simulink model "Longitudinal_new"  (R2025b)
settings: Solver=VariableStepAuto  StartTime=0.0  StopTime=5  MaxStep=0.001  RelTol=1e-3
undefined symbols (not defined in the file): car, rad, s, Tau_1, Tau_2, Tau_3, Tau_4, Tau_EM, tyre
libraries: aerolibconvert2 x7, simulink x4, autolibcoupling x2
(part 3 of 3)

== matlab function Longitudinal_new/longitudinal dynamics/Kinematics/FL/Front Left Tyre ==
  data: car input; wheel_travel_FL output; IR_FL input; AD_FL input; Fz_FL input; h_ground_FL output; delta_Fz input; delta_z_tyre_FL output; a input
function [wheel_travel_FL, h_ground_FL, delta_z_tyre_FL] = kinematics(car, IR_FL, AD_FL, Fz_FL, delta_Fz, a)

delta_z_tyre_FL = Fz_FL / car.k_tyre/1000; % tyre vertical stiffness - kz_tyre - for front and rear tyres, look at buses
k_spring_ground_FL = (car.k_spring_front * IR_FL^2) + car.k_flexure;

if a > 0 % under acceleration
    delta_z_spring_FL = Fz_FL / k_spring_ground_FL; % front axle
else % under braking
    delta_z_spring_FL = (Fz_FL - delta_Fz) / k_spring_ground_FL + delta_Fz * ((1-AD_FL/100)/k_spring_ground_FL) ; % front axle
end

%wheel center movement only due to spring deflection at ground. 
%to be used in the kineamtics block (camber, antidive, ir,...)
wheel_travel_FL = delta_z_spring_FL - car.z0_spring_front; % if negative it is bounce

%to be used to find the new height of the car from the ground
jounce_FL = delta_z_tyre_FL + delta_z_spring_FL - car.z0_front;
h_ground_FL = car.h0_ground_front - jounce_FL;

== matlab function Longitudinal_new/longitudinal dynamics/slip_tyres/FR ==
  data: delta_Fx_front input; delta_z_tyre_FR input; w_dot_slip_FR output; car input
function w_dot_slip_FR  = slip(delta_Fx_front, delta_z_tyre_FR, car)


    w_dot_slip_FR = (delta_Fx_front * (car.R - delta_z_tyre_FR)) / car.J_f; %rad/s^2

== matlab function Longitudinal_new/Tyres1/Rear Left ==
  data: car input; Fx_RL output; SR input; Fz input; camber input
function Fx_RL = fcn(car,SR,Fz,camber)

% PAC2002 puro longitudinale (Fx vs k)

     Fz0 = car.tyre_Fz0;
     if Fz0 == 0, Fz0 = max(1, Fz); end
    dfz = (Fz - Fz0)/Fz0;

    pi0 = car.tyre_pi0;  % Pa nominale
    dpi = (car.tyre_pressure_rear - pi0)/pi0;
    
Cx1 = car.tyre_Cx1;
Dx1 = car.tyre_Dx1;
Dx2 = car.tyre_Dx2;
Dx3 = car.tyre_Dx3;
Ex1 = car.tyre_Ex1;
Ex2 = car.tyre_Ex2;
Ex3 = car.tyre_Ex3;
Ex4 = car.tyre_Ex4;
Kx1 = car.tyre_Kx1;
Kx2 = car.tyre_Kx2;
Kx3 = car.tyre_Kx3;
Hx1 = car.tyre_Hx1;
Hx2 = car.tyre_Hx2;
Vx1 = car.tyre_Vx1;
Vx2 = car.tyre_Vx2;
px1 = car.tyre_px1;
px2 = car.tyre_px2;
px3 = car.tyre_px3;
px4 = car.tyre_px4;
% lmux = car.tyre_lmux;


    gamma = camber*pi/180;
    mu = (Dx1 + Dx2*dfz) * (1 - Dx3*(gamma^2)) * (1 + px3*dpi + px4*dpi^2)*car.scale_factor;
    % mu = 1.4;

    D = mu * Fz;
    C = Cx1;
    K = Fz * (Kx1 + Kx2*dfz) * exp(Kx3*dfz) * (1 + px1*dpi + px2*dpi^2);
    B = K / (C*D + eps);

    SH = Hx1 + Hx2*dfz;
    SR  = SR + SH;

    E  = (Ex1 + Ex2*dfz + Ex3*dfz^2) * (1 - Ex4*sign(SR));
    SV = Fz * (Vx1 + Vx2*dfz);

    Fx0 = D * sin( C * atan( B*SR - E*(B*SR - atan(B*SR)) ) );
    Fx_RL = Fx0 + SV;

== matlab function Longitudinal_new/Tyres1/Rear Right ==
  data: car input; Fx_RR output; SR input; Fz input; camber input
function Fx_RR = fcn(car,SR,Fz,camber)

% PAC2002 puro longitudinale (Fx vs k)

     Fz0 = car.tyre_Fz0;
     if Fz0 == 0, Fz0 = max(1, Fz); end
    dfz = (Fz - Fz0)/Fz0;

    pi0 = car.tyre_pi0;  % Pa nominale
    dpi = (car.tyre_pressure_rear - pi0)/pi0;
    
Cx1 = car.tyre_Cx1;
Dx1 = car.tyre_Dx1;
Dx2 = car.tyre_Dx2;
Dx3 = car.tyre_Dx3;
Ex1 = car.tyre_Ex1;
Ex2 = car.tyre_Ex2;
Ex3 = car.tyre_Ex3;
Ex4 = car.tyre_Ex4;
Kx1 = car.tyre_Kx1;
Kx2 = car.tyre_Kx2;
Kx3 = car.tyre_Kx3;
Hx1 = car.tyre_Hx1;
Hx2 = car.tyre_Hx2;
Vx1 = car.tyre_Vx1;
Vx2 = car.tyre_Vx2;
px1 = car.tyre_px1;
px2 = car.tyre_px2;
px3 = car.tyre_px3;
px4 = car.tyre_px4;
% lmux = car.tyre_lmux;


    gamma = camber*pi/180;
    mu = (Dx1 + Dx2*dfz) * (1 - Dx3*(gamma^2)) * (1 + px3*dpi + px4*dpi^2)*car.scale_factor;
    % mu = 1.4;

    D = mu * Fz;
    C = Cx1;
    K = Fz * (Kx1 + Kx2*dfz) * exp(Kx3*dfz) * (1 + px1*dpi + px2*dpi^2);
    B = K / (C*D + eps);

    SH = Hx1 + Hx2*dfz;
    SR  = SR + SH;

    E  = (Ex1 + Ex2*dfz + Ex3*dfz^2) * (1 - Ex4*sign(SR));
    SV = Fz * (Vx1 + Vx2*dfz);

    Fx0 = D * sin( C * atan( B*SR - E*(B*SR - atan(B*SR)) ) );
    Fx_RR = Fx0 + SV;

== matlab function Longitudinal_new/Powertrain/MATLAB Function ==
  settings: updateMethod=DISCRETE
  data: T_RL_in input; T_RR_in input; T_RL_out output; trigger input; T_RR_out output; time input
function [T_RL_out,T_RR_out] = fcn(T_RL_in, T_RR_in, trigger, time)

persistent t_start is_active prev_trigger
if isempty(t_start)
    t_start     = 0;
    is_active   = false;
    prev_trigger = 0;
end

% Rileva fronte di salita del trigger
if trigger == 1 && prev_trigger == 0
    t_start   = time;     % istante in cui parte il taglio coppia
    is_active = true;
end

% Disattiva dopo 0.15 s
if is_active && (time - t_start >= 0.15)
    is_active = false;
end

% Aggiorna trigger precedente
prev_trigger = trigger;

% Logica di uscita
if is_active
    T_RL_out = 0;
    T_RR_out = 0;
else
    T_RL_out = T_RL_in;
    T_RR_out = T_RR_in;
end
end

== matlab function Longitudinal_new/Powertrain/Clutch/MATLAB Function ==
  data: threshold input; w_out output; w_rear_in input; w_rear_out output
function [w_out, w_rear_out] = fcn(threshold, w_rear_in)

if w_rear_in < threshold
    w_out=threshold;
    w_rear_out=0;
else
    w_out=0;
    w_rear_out=w_rear_in;
end

== matlab function Longitudinal_new/longitudinal dynamics/Jr/MATLAB Function ==
  data: gear input; Jr_tot output; car input
function Jr_tot  = Jr(gear, car)

if gear == 1 
    Jr_tot = car.Jr_tot_1;
elseif gear == 2 
    Jr_tot = car.Jr_tot_2;
elseif gear == 3 
    Jr_tot = car.Jr_tot_3;
elseif gear == 4
    Jr_tot = car.Jr_tot_4;
else  
    Jr_tot = car.Jr_tot_0;
end

== matlab function Longitudinal_new/Powertrain/Clutch/MATLAB Function1 ==
  data: threshold input; w_out output; w_rear_in input; w_rear_out output
function [w_out, w_rear_out] = fcn(threshold, w_rear_in)

persistent isZero   % flag that stays true once threshold is reached

% Initialize the flag the first time the function is called
if isempty(isZero)
    isZero = false;
end

if w_rear_in >= threshold
    isZero = true;
end

% Output logic
if isZero
    w_out = 0;
    w_rear_out = w_rear_in;
else
    w_out = threshold;
    w_rear_out = 0;
end

end

== matlab function Longitudinal_new/Powertrain1/Driver model - gear selection1/MATLAB Function3 ==
  settings: updateMethod=DISCRETE
  data: gear_trigger output; car input; gear_out output; v input
function [gear_trigger, gear_out] = change_gear(car, v)

    persistent gear
    if isempty(gear)
        gear = 2;      % start in 2nd
    end

    R = car.R; %

    % thresholds
    v_thresh_up   = [0, 24.9444, 45];   % 1-2, 2-3, 3-4
    % v_thresh_down = [0, 15, 15];          % 2-1, 3-2, 4-3, i numeri sono a caso quindi da cambiare

    tau      = [13.8304, 9.9320, 8.5118, 7.4490];
    nGearMax = numel(tau);

    gear_trigger = 0;
    old_gear     = gear;   % save old gear
    gear_out     = old_gear;

    % - UPSHIFT
    if old_gear < nGearMax && v >= v_thresh_up(old_gear)
        gear = old_gear + 1;
        gear_trigger = 1;

    % % - DOWNSHIFT
    % elseif old_gear > 2 && v <= v_thresh_down(old_gear)
    %     gear = old_gear - 1;
    %     gear_trigger = -1;
    % end

    gear_out = gear;
end

== matlab function Longitudinal_new/longitudinal dynamics/Fx powertrain calculation/RR ==
  data: Fx_ICE_RR output; T input; T_b input; a input; Fz input; J_r input; car input; delta_z_tyre_RR input
function Fx_ICE_RR = fcn( T, T_b,a, Fz, J_r, car, delta_z_tyre_RR)

Fx_ICE_RR = ( T - T_b - Fz * car.delta - J_r * a / ( car.R - delta_z_tyre_RR ) ) / ( car.R - delta_z_tyre_RR ) ; %N; % J - parameter for each tyre - J_f & J_r

== matlab function Longitudinal_new/longitudinal dynamics/Fx powertrain calculation/FR ==
  data: Fx_EM_FR output; T input; T_b input; Fz input; a input; car input; delta_z_tyre_FR input
function Fx_EM_FR = fcn( T, T_b,Fz, a, car, delta_z_tyre_FR )

Fx_EM_FR = ( T - T_b - Fz * car.delta - car.J_f * a / ( car.R - delta_z_tyre_FR ) ) / ( car.R - delta_z_tyre_FR ) ; %N % J - parameter for each tyre - J_f & J_r

== matlab function Longitudinal_new/Tyres1/Front Left ==
  data: car input; Fx_FL output; SR input; Fz input; camber input
function Fx_FL = fcn(car,SR,Fz,camber)

% PAC2002 puro longitudinale (Fx vs k)

     Fz0 = car.tyre_Fz0;
     if Fz0 == 0, Fz0 = max(1, Fz); end
    dfz = (Fz - Fz0)/Fz0;

    pi0 = car.tyre_pi0;  % Pa nominale
    dpi = (car.tyre_pressure_front - pi0)/pi0;
    
Cx1 = car.tyre_Cx1;
Dx1 = car.tyre_Dx1;
Dx2 = car.tyre_Dx2;
Dx3 = car.tyre_Dx3;
Ex1 = car.tyre_Ex1;
Ex2 = car.tyre_Ex2;
Ex3 = car.tyre_Ex3;
Ex4 = car.tyre_Ex4;
Kx1 = car.tyre_Kx1;
Kx2 = car.tyre_Kx2;
Kx3 = car.tyre_Kx3;
Hx1 = car.tyre_Hx1;
Hx2 = car.tyre_Hx2;
Vx1 = car.tyre_Vx1;
Vx2 = car.tyre_Vx2;
px1 = car.tyre_px1;
px2 = car.tyre_px2;
px3 = car.tyre_px3;
px4 = car.tyre_px4;
% lmux = car.tyre_lmux;


    gamma = camber*pi/180;
    mu = (Dx1 + Dx2*dfz) * (1 - Dx3*(gamma^2)) * (1 + px3*dpi + px4*dpi^2)*car.scale_factor;
    % mu = 1.4;

    D = mu * Fz;
    C = Cx1;
    K = Fz * (Kx1 + Kx2*dfz) * exp(Kx3*dfz) * (1 + px1*dpi + px2*dpi^2);
    B = K / (C*D + eps);

    SH = Hx1 + Hx2*dfz;
    SR  = SR + SH;

    E  = (Ex1 + Ex2*dfz + Ex3*dfz^2) * (1 - Ex4*sign(SR));
    SV = Fz * (Vx1 + Vx2*dfz);

    Fx0 = D * sin( C * atan( B*SR - E*(B*SR - atan(B*SR)) ) );
    Fx_FL = Fx0 + SV;

== matlab function Longitudinal_new/longitudinal dynamics/Fx powertrain calculation/RL ==
  data: T input; T_b input; Fz input; a input; J_r input; car input; Fx_ICE_RL output; delta_z_tyre_RL input
function Fx_ICE_RL = fcn( T, T_b, Fz, a, J_r, car, delta_z_tyre_RL)

Fx_ICE_RL = ( T - T_b - Fz * car.delta - J_r * a / ( car.R - delta_z_tyre_RL ) ) / ( car.R - delta_z_tyre_RL ) ; %N % J - parameter for each tyre - J_f & J_r

== matlab function Longitudinal_new/longitudinal dynamics/delta_ Fx solver/RL ==
  data: Fx_ICE input; Fx_tyre input; delta_Fx_RL output
function delta_Fx_RL  = fcn(Fx_ICE, Fx_tyre)

delta_Fx_RL = Fx_ICE - Fx_tyre;

== matlab function Longitudinal_new/longitudinal dynamics/delta_ Fx solver/FR ==
  data: Fx_EM input; Fx_tyre input; delta_Fx_FR output
function delta_Fx_FR  = fcn(Fx_EM, Fx_tyre)

delta_Fx_FR = Fx_EM - Fx_tyre ;

== matlab function Longitudinal_new/longitudinal dynamics/delta_ Fx solver/FL ==
  data: Fx_EM input; Fx_tyre input; delta_Fx_FL output
function delta_Fx_FL  = fcn(Fx_EM, Fx_tyre)

delta_Fx_FL = Fx_EM - Fx_tyre;

== matlab function Longitudinal_new/Powertrain/Driver model - gear selection/MATLAB Function3 ==
  settings: updateMethod=DISCRETE
  data: gear_trigger output; car input; gear_out output; v input
function [gear_trigger, gear_out] = change_gear(car, v)

    persistent gear
    if isempty(gear)
        gear = 2;      % start in 2nd
    end

    R = car.R; %

    % thresholds
    v_thresh_up   = [0, 24.9444, 45];   % 1-2, 2-3, 3-4
    v_thresh_down = [0, 15, 15];          % 2-1, 3-2, 4-3, i numeri sono a caso quindi da cambiare

    tau      = [13.8304, 9.9320, 8.5118, 7.4490];
    nGearMax = numel(tau);

    gear_trigger = 0;
    old_gear     = gear;   % save old gear
    gear_out     = old_gear;

    % - UPSHIFT
    if old_gear < nGearMax && v >= v_thresh_up(old_gear)
        gear = old_gear + 1;
        gear_trigger = 1;

    % - DOWNSHIFT
    elseif old_gear > 2 && v <= v_thresh_down(old_gear)
        gear = old_gear - 1;
        gear_trigger = -1;
    end

    gear_out = gear;
end

== matlab function Longitudinal_new/longitudinal dynamics/slip_tyres/FL ==
  data: delta_Fx_front input; delta_z_tyre_FL input; w_dot_slip_FL output; car input
function w_dot_slip_FL  = slip(delta_Fx_front, delta_z_tyre_FL, car)

w_dot_slip_FL = delta_Fx_front * (car.R - delta_z_tyre_FL) / car.J_f;

== matlab function Longitudinal_new/longitudinal dynamics/slip_tyres/RL ==
  data: delta_Fx_rear input; w_dot_slip_RL output; delta_z_tyre_RL input; J_r input; car input
function w_dot_slip_RL  = slip(delta_Fx_rear, delta_z_tyre_RL, J_r, car)

w_dot_slip_RL = delta_Fx_rear * (car.R - delta_z_tyre_RL) / ( J_r );

== matlab function Longitudinal_new/Powertrain1/MATLAB Function2 ==
  data: w_ICE input; T_powertrain output; T_ICE input; w_rear input; T_clutch input; abs_w output
function [T_powertrain, abs_w] = Clutch(w_ICE, T_ICE, w_rear, T_clutch)

abs_w = w_ICE - w_rear;

if abs_w < 50
    T_powertrain = T_ICE;
else 
    T_powertrain = T_clutch;
end

== matlab function Longitudinal_new/Powertrain1/Clutch/MATLAB Function ==
  data: threshold input; w_out output; w_rear_in input; w_rear_out output
function [w_out, w_rear_out] = fcn(threshold, w_rear_in)

if w_rear_in < threshold
    w_out=threshold;
    w_rear_out=0;
else
    w_out=0;
    w_rear_out=w_rear_in;
end

== matlab function Longitudinal_new/Powertrain1/Clutch/MATLAB Function1 ==
  data: threshold input; w_out output; w_rear_in input; w_rear_out output
function [w_out, w_rear_out] = fcn(threshold, w_rear_in)

persistent isZero   % flag that stays true once threshold is reached

% Initialize the flag the first time the function is called
if isempty(isZero)
    isZero = false;
end

if w_rear_in >= threshold
    isZero = true;
end

% Output logic
if isZero
    w_out = 0;
    w_rear_out = w_rear_in;
else
    w_out = threshold;
    w_rear_out = 0;
end

end

== matlab function Longitudinal_new/longitudinal dynamics/Fx equilibrium ==
  data: Drag output; Fz_FL output; a input; Fz_RR output; Fz_RL output; Fz_FR output; delta_Fz output; v input; Cx input; Cz input; delta_wb_front input; delta_wb_rear input; Jr_tot input; car input
function [Drag, Fz_FL, Fz_RR, Fz_RL, Fz_FR, delta_Fz] = fx_equilibrium(a, v, Cx, Cz, delta_wb_front, delta_wb_rear, Jr_tot, car)

wb = car.wb0 + delta_wb_front + delta_wb_rear; %m

Downforce = 0.5 * car.rho * Cz * car.frontal_area * v ^ 2; % downforce N
Drag = 0.5 * car.rho * Cx * car.frontal_area * v ^ 2; % drag N
M_aero = Drag * (car.h_cp - car.h_cog) - Downforce * (car.lf - car.x_cp); %Nm

delta_Fz = car.m * a * car.h_cog / wb + Drag * car.h_cog / wb + M_aero / wb; %N
delta_Fz=delta_Fz/2;
%J_f è di una singola ruota
%J_r totale da ruota a motore ICE
Fz_front = -(car.m * a + Drag) * car.h_cog / wb + (car.m * car.g + Downforce) * (car.lr + delta_wb_rear - car.delta) / wb - M_aero / wb - car.J_f*2* a / (car.R * wb); %N  (verificare J_f*4 oppure J_f*2!!!!!!!!!!!)

Fz_rear = (car.m * a + Drag) * car.h_cog / wb + (car.m * car.g + Downforce) * (car.lf + delta_wb_front + car.delta) / wb + M_aero / wb + Jr_tot * a / (car.R * wb); %N

if Fz_front <= 0
    Fz_rear = Fz_rear + Fz_front;
    Fz_front = 0;
elseif Fz_rear <0 
    Fz_front = Fz_front + Fz_rear;
    Fz_rear = 0;
end

Fz_FR = Fz_front / 2 ;
Fz_FL = Fz_FR ;

Fz_RL = Fz_rear / 2;
Fz_RR = Fz_RL ;

== matlab function Longitudinal_new/Powertrain1/Driver model - gear selection/MATLAB Function3 ==
  settings: updateMethod=DISCRETE
  data: gear_trigger output; car input; gear_out output; v input
function [gear_trigger, gear_out] = change_gear(car, v)

    persistent gear
    if isempty(gear)
        gear = 2;      % start in 2nd
    end

    R = car.R; %

    % thresholds
    v_thresh_up   = [0, 24.9444, 45];   % 1-2, 2-3, 3-4
    v_thresh_down = [0, 15, 15];          % 2-1, 3-2, 4-3, i numeri sono a caso quindi da cambiare

    tau      = [13.8304, 9.9320, 8.5118, 7.4490];
    nGearMax = numel(tau);

    gear_trigger = 0;
    old_gear     = gear;   % save old gear
    gear_out     = old_gear;

    % - UPSHIFT
    if old_gear < nGearMax && v >= v_thresh_up(old_gear)
        gear = old_gear + 1;
        gear_trigger = 1;

    % - DOWNSHIFT
    elseif old_gear > 2 && v <= v_thresh_down(old_gear)
        gear = old_gear - 1;
        gear_trigger = -1;
    end

    gear_out = gear;
end

== matlab function Longitudinal_new/Powertrain1/MATLAB Function ==
  settings: updateMethod=DISCRETE
  data: T_RL_in input; T_RR_in input; T_RL_out output; trigger input; T_RR_out output; time input
function [T_RL_out,T_RR_out] = fcn(T_RL_in, T_RR_in, trigger, time)

persistent t_start is_active prev_trigger
if isempty(t_start)
    t_start     = 0;
    is_active   = false;
    prev_trigger = 0;
end

% Rileva fronte di salita del trigger
if trigger == 1 && prev_trigger == 0
    t_start   = time;     % istante in cui parte il taglio coppia
    is_active = true;
end

% Disattiva dopo 0.15 s
if is_active && (time - t_start >= 0.15)
    is_active = false;
end

% Aggiorna trigger precedente
prev_trigger = trigger;

% Logica di uscita
if is_active
    T_RL_out = 0;
    T_RR_out = 0;
else
    T_RL_out = T_RL_in;
    T_RR_out = T_RR_in;
end
end

== matlab function Longitudinal_new/Powertrain1/MATLAB Function1 ==
  settings: updateMethod=DISCRETE
  data: T_RL_in input; T_RR_in input; T_RL_out output; trigger input; T_RR_out output; time input
function [T_RL_out,T_RR_out] = fcn(T_RL_in, T_RR_in, trigger, time)

persistent t_start is_active prev_trigger
if isempty(t_start)
    t_start     = 0;
    is_active   = false;
    prev_trigger = 0;
end

% Rileva fronte di salita del trigger
if trigger == 1 && prev_trigger == 0
    t_start   = time;     % istante in cui parte il taglio coppia
    is_active = true;
end

% Disattiva dopo 0.15 s
if is_active && (time - t_start >= 0.15)
    is_active = false;
end

% Aggiorna trigger precedente
prev_trigger = trigger;

% Logica di uscita
if is_active
    T_RL_out = 0;
    T_RR_out = 0;
else
    T_RL_out = T_RL_in;
    T_RR_out = T_RR_in;
end
end

== matlab function Longitudinal_new/longitudinal dynamics/Fx powertrain calculation/FL ==
  data: Fx_EM_FL output; T input; T_b input; Fz input; a input; car input; delta_z_tyre_FL input
function Fx_EM_FL = fcn( T,T_b, Fz, a, car, delta_z_tyre_FL)

Fx_EM_FL = ( T - T_b - Fz * car.delta - car.J_f * a / ( car.R - delta_z_tyre_FL ) ) / ( car.R - delta_z_tyre_FL ) ; %N
% J - parameter for each tyre - J_f & J_r

== matlab function Longitudinal_new/Tyres/Rear Right ==
  data: tyre_RR input; Fx output; Fy output
function [Fx, Fy] = fcn(tyre_RR)

y = u;

== matlab function Longitudinal_new/Tyres/Front Right ==
  data: SR input; tyre input; Fx output; p input; Fz input; camber input
function Fx = fcn(SR,tyre,p,Fz,camber)

% PAC2002 puro longitudinale (Fx vs k)

     Fz0 = tyre.Fz0;
     if Fz0 == 0, Fz0 = max(1, Fz); end
    dfz = (Fz - Fz0)/Fz0;

    pi0 = tyre.pi0;  % Pa nominale
    dpi = (p - pi0)/pi0;
    
    Cx1 = tyre.Cx1;
    Dx1 = tyre.Dx1;
    Dx2 = tyre.Dx2;
    Dx3 = tyre.Dx3;
    Ex1 = tyre.Ex1;
    Ex2 = tyre.Ex2;
    Ex3 = tyre.Ex3;
    Ex4 = tyre.Ex4;
    Kx1 = tyre.Kx1;
    Kx2 = tyre.Kx2;
    Kx3 = tyre.Kx3;
    Hx1 = tyre.Hx1;
    Hx2 = tyre.Hx2;
    Vx1 = tyre.Vx1;
    Vx2 = tyre.Vx2;
    px1 = tyre.px1;
    px2 = tyre.px2;
    px3 = tyre.px3;
    px4 = tyre.px4;
    lmux = tyre.lmux;

    gamma = camber*pi/180;
    mu = (Dx1 + Dx2*dfz) * (1 - Dx3*(gamma^2)) * (1 + px3*dpi + px4*dpi^2)*lmux;
    % mu = 1.4;

    D = mu * Fz;
    C = Cx1;
    K = Fz * (Kx1 + Kx2*dfz) * exp(Kx3*dfz) * (1 + px1*dpi + px2*dpi^2);
    B = K / (C*D + eps);

    SH = Hx1 + Hx2*dfz;
    SR  = SR + SH;

    E  = (Ex1 + Ex2*dfz + Ex3*dfz^2) * (1 - Ex4*sign(SR));
    SV = Fz * (Vx1 + Vx2*dfz);

    Fx0 = D * sin( C * atan( B*SR - E*(B*SR - atan(B*SR)) ) );
    Fx = Fx0 + SV;

== matlab function Longitudinal_new/Tyres/Rear Left ==
  data: tyre_RL input; Fx output; Fy output
function [Fx, Fy] = fcn(tyre_RL)

y = u;

== matlab function Longitudinal_new/longitudinal dynamics/Kinematics/RL/Rear Left Tyre ==
  data: car input; wheel_travel_RL output; IR_RL input; AS_RL input; Fz_RL input; h_ground_RL output; delta_Fz input; delta_z_tyre_RL output; a input
function [wheel_travel_RL, h_ground_RL, delta_z_tyre_RL]      = kinematics(car, IR_RL, AS_RL, Fz_RL, delta_Fz, a)

delta_z_tyre_RL = Fz_RL / car.k_tyre/1000; % tyre vertical stiffness - kz_tyre - for front and rear tyres, look at buses
k_spring_ground_RL = (car.k_spring_rear * IR_RL^2);

if a > 0 % under acceleration
    delta_z_spring_RL = (Fz_RL - delta_Fz) / k_spring_ground_RL + delta_Fz * ((1-AS_RL/100)/k_spring_ground_RL) ; % rear axle
else % under braking
    delta_z_spring_RL = Fz_RL / k_spring_ground_RL; % rear axle
end

%wheel center movement only due to spring deflection at ground. 
%to be used in the kineamtics block (camber, antidive, ir,...)
wheel_travel_RL = delta_z_spring_RL - car.z0_spring_rear; % if negative it is bounce

%to be used to find the new height of the car from the ground
jounce_RL = delta_z_tyre_RL + delta_z_spring_RL - car.z0_rear;
h_ground_RL = car.h0_ground_rear - jounce_RL;
